simulink model "d_anderson_farmer"  (Simulink 5.1)
settings: Solver=ode45  StartTime=0.0  StopTime=10.0  RelTol=1e-3
libraries: fm_lib x1
(part 1 of 2)
settings Model: Creator=fmilano  LastModifiedBy=fmilano  ExtModeAutoUpdateStatusClock=off  SignalLoggingName=logsout  BooleanDataType=on  RTWOptions="-aEnforceIntegerDowncast=1 -aFoldNonRolledExpr=1 -aInlineInvariantSignals=0 -aInlineParameters=0 -aLocalBlockOutputs=1 -aRollThreshold=5 -aZeroInternalMemoryAtStartup=1 -aZeroExternalMemoryAtStartup=1 -aInitFltsAndDblsToZero=1 -aForceBlockIOInitOptimize=0 -aGenerateReport=0 -aGenCodeOnly=0 -aRTWVerbose=1 -aIncludeHyperlinkInReport=0 -aLaunchReport=0 -aGenerateTraceInfo=0  -aForceParamTrailComments=0 -aGenerateComments=1 -aIgnoreCustomStorageClasses=1 -aIncHierarchyInIds=0 -aMaxRTWIdLen=31 -aShowEliminatedStatements=0 -aIncDataTypeInIds=0 -aInsertBlockDesc=0 -aIgnoreTestpoints=0 -aSimulinkBlockComments=1 -aInlinedPrmAccess=\"Literals\"  -aSuppressErrorStatus=0 -aModelReferenceCompliant=1 -aParenthesesLevel=\"Nominal\" -aModelStepFunctionPrototypeControlCompliant=0 -aPortableWordSizes=0 -aParMdlRefBuildCompliant=1 -aSupportNonInlinedSFcns=1 -aSupportContinuousTime=1 -aSupportComplex=1 -aSupportNonFinite=1 -aSupportAbsoluteTime=1 -aMultiwordLength=2048 -aTargetPreCompLibLocation=\"\" -aTargetLibSuffix=\"\" -aTargetFunctionLibrary=\"ANSI_C\" -aTargetFcnLib=\"ansi_tfl_tmw.mat\" -aMultiInstanceERTCode=0 -aLogVarNameModifier=\"rt_\" -aERTFirstTimeCompliant=0 -aIsPILTarget=0 -aCombineOutputUpdateFcns=0 -aGenerateASAP2=0 -aGenerateClassInterface=0 -aGenerateTestInterfaces=0 -aGenerateSampleERTMain=0 -aGenerateFullHeader=1 -aUtilityFuncGeneration=\"Auto\" -aIncludeFileDelimiter=\"Auto\" -aIncludeMdlTerminateFcn=1 -aPurelyIntegerCode=0 -aAutosarCompliant=0 -aERTCustomFileBanners=0 -aRTWCAPIStates=0 -aRTWCAPIParams=0 -aRTWCAPISignals=0 -aMatFileLogging=1 -aCompOptLevelCompliant=0 -aCPPClassGenCompliant=0 -aExtModeIntrfLevel=\"Level1\" -aExtModeMexFile=\"ext_comm\" -aExtModeTransport=0 -aExtModeStaticAllocSize=1000000 -aExtModeTesting=0 -aExtModeStaticAlloc=0 -aExtMode=0 -aERTMultiwordLength=256 -aERTMultiwordTypeDef=\"System defined\"  -aGenerateTraceInfo=0 -aGenerateTraceInfo=0 -aGenerateTraceInfo=0 -aGenerateTraceInfo=0 -aPrefixModelToSubsysFcnNames=1"

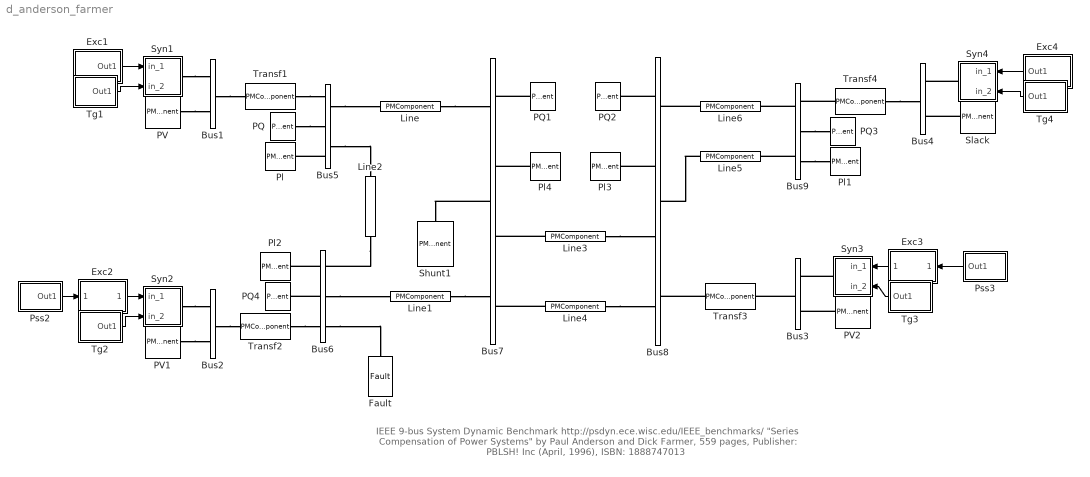
== system d_anderson_farmer ==
  note: IEEE 9-bus System Dynamic Benchmark
      |
      | http://psdyn.ece.wisc.edu/IEEE_benchmarks/
      |
      | "Series Compensation of Power Systems" by Paul Anderson and Dick Farmer,
      | 559 pages, Publisher: PBLSH! Inc (April, 1996), ISBN: 1888747013
  Bus1 : PMComponent  Tag=PSATblock  Description=Connection  PhysicalDomain=psatdomain  LeftPortType=p1  RightPortType=p1  LConnTagsString=__newl0|__newl1  RConnTagsString=__newr0  mask(Bus){in=2, out=1, p2q=20, p3_4q=[1.00   0.00], p5q=2, p6q=1}
      mask prompts: in "Number of inputs:"; out "Number of outputs:"; p2q "Voltage Rating [kV]"; p3_4q "Voltage initial guess [p.u.   rad]"; p5q "Area number"; p6q "Region number"
      mask help: Bus block
      mask init:
      | fm_inout
      settings: AttributesFormatString="|V| =  1.03   p.u.\\n<V  =  0.1540 rad"
      mask CallbackString: ||||fm_block|
      mask Display: plot([0 1 1 0 0],[0 0 1 1 0])
  Bus2 : PMComponent  Tag=PSATblock  Description=Connection  PhysicalDomain=psatdomain  LeftPortType=p1  RightPortType=p1  LConnTagsString=__newl0|__newl1  RConnTagsString=__newr0  mask(Bus){in=2, out=1, p2q=20, p3_4q=[1.00   0.00], p5q=1, p6q=1}
      mask prompts: in "Number of inputs:"; out "Number of outputs:"; p2q "Voltage Rating [kV]"; p3_4q "Voltage initial guess [p.u.   rad]"; p5q "Area number"; p6q "Region number"
      mask help: Bus block
      mask init:
      | fm_inout
      settings: AttributesFormatString="|V| =  1.05   p.u.\\n<V  =  0.1208 rad"
      mask CallbackString: ||||fm_block|
      mask Display: plot([0 1 1 0 0],[0 0 1 1 0])
  Bus3 : PMComponent  Tag=PSATblock  Description=Connection  PhysicalDomain=psatdomain  LeftPortType=p1  RightPortType=p1  LConnTagsString=__newl0  RConnTagsString=__newr0|__newr1  mask(Bus){in=1, out=2, p2q=20, p3_4q=[1.00   0.00], p5q=1, p6q=1}
      mask prompts: in "Number of inputs:"; out "Number of outputs:"; p2q "Voltage Rating [kV]"; p3_4q "Voltage initial guess [p.u.   rad]"; p5q "Area number"; p6q "Region number"
      mask help: Bus block
      mask init:
      | fm_inout
      settings: AttributesFormatString="|V| =  1.032  p.u.\\n<V  =  0.3131 rad"
      mask CallbackString: ||||fm_block|
      mask Display: plot([0 1 1 0 0],[0 0 1 1 0])
  Bus4 : PMComponent  Tag=PSATblock  Description=Connection  PhysicalDomain=psatdomain  LeftPortType=p1  RightPortType=p1  LConnTagsString=__newl0  RConnTagsString=__newr0|__newr1  mask(Bus){in=1, out=2, p2q=20, p3_4q=[1.00   0.00], p5q=3, p6q=1}
      mask prompts: in "Number of inputs:"; out "Number of outputs:"; p2q "Voltage Rating [kV]"; p3_4q "Voltage initial guess [p.u.   rad]"; p5q "Area number"; p6q "Region number"
      mask help: Bus block
      mask init:
      | fm_inout
      settings: AttributesFormatString="|V| =  1.02   p.u.\\n<V  =  0      rad"
      mask CallbackString: ||||fm_block|
      mask Display: plot([0 1 1 0 0],[0 0 1 1 0])
  Bus5 : PMComponent  Tag=PSATblock  Description=Connection  PhysicalDomain=psatdomain  LeftPortType=p1  RightPortType=p1  LConnTagsString=__newl0|__newl1|__newl2  RConnTagsString=__newr0|__newr1  mask(Bus){in=3, out=2, p2q=400, p3_4q=[1.00   0.00], p5q=2, p6q=1}
      mask prompts: in "Number of inputs:"; out "Number of outputs:"; p2q "Voltage Rating [kV]"; p3_4q "Voltage initial guess [p.u.   rad]"; p5q "Area number"; p6q "Region number"
      mask help: Bus block
      mask init:
      | fm_inout
      settings: AttributesFormatString="|V| =  1.0118 p.u.\\n<V  =  0.0752 rad"
      mask CallbackString: ||||fm_block|
      mask Display: plot([0 1 1 0 0],[0 0 1 1 0])
  Bus6 : PMComponent  Tag=PSATblock  Description=Connection  PhysicalDomain=psatdomain  LeftPortType=p1  RightPortType=p1  LConnTagsString=__newl0|__newl1|__newl2  RConnTagsString=__newr0|__newr1|__newr2  mask(Bus){in=3, out=3, p2q=400, p3_4q=[1.00   0.00], p5q=1, p6q=1}
      mask prompts: in "Number of inputs:"; out "Number of outputs:"; p2q "Voltage Rating [kV]"; p3_4q "Voltage initial guess [p.u.   rad]"; p5q "Area number"; p6q "Region number"
      mask help: Bus block
      mask init:
      | fm_inout
      settings: AttributesFormatString="|V| =  1.0397 p.u.\\n<V  =  0.0481 rad"
      mask CallbackString: ||||fm_block|
      mask Display: plot([0 1 1 0 0],[0 0 1 1 0])
  Bus7 : PMComponent  Tag=PSATblock  Description=Connection  PhysicalDomain=psatdomain  LeftPortType=p1  RightPortType=p1  LConnTagsString=__newl0|__newl1|__newl2  RConnTagsString=__newr0|__newr1|__newr2|__newr3  mask(Bus){in=3, out=4, p2q=400, p3_4q=[1.00   0.00], p5q=1, p6q=1}
      mask prompts: in "Number of inputs:"; out "Number of outputs:"; p2q "Voltage Rating [kV]"; p3_4q "Voltage initial guess [p.u.   rad]"; p5q "Area number"; p6q "Region number"
      mask help: Bus block
      mask init:
      | fm_inout
      settings: AttributesFormatString="|V| =  1.0209 p.u.\\n<V  = -0.1371 rad"
      mask CallbackString: ||||fm_block|
      mask Display: plot([0 1 1 0 0],[0 0 1 1 0])
  Bus8 : PMComponent  Tag=PSATblock  Description=Connection  PhysicalDomain=psatdomain  LeftPortType=p1  RightPortType=p1  LConnTagsString=__newl0|__newl1|__newl2|__newl3  RConnTagsString=__newr0|__newr1|__newr2  mask(Bus){in=4, out=3, p2q=400, p3_4q=[1.00   0.00], p5q=1, p6q=1}
      mask prompts: in "Number of inputs:"; out "Number of outputs:"; p2q "Voltage Rating [kV]"; p3_4q "Voltage initial guess [p.u.   rad]"; p5q "Area number"; p6q "Region number"
      mask help: Bus block
      mask init:
      | fm_inout
      settings: AttributesFormatString="|V| =  1.0247 p.u.\\n<V  =  0.2415 rad"
      mask CallbackString: ||||fm_block|
      mask Display: plot([0 1 1 0 0],[0 0 1 1 0])
  Bus9 : PMComponent  Tag=PSATblock  Description=Connection  PhysicalDomain=psatdomain  LeftPortType=p1  RightPortType=p1  LConnTagsString=__newl0|__newl1  RConnTagsString=__newr0|__newr1|__newr2  mask(Bus){in=2, out=3, p2q=400, p3_4q=[1.00   0.00], p5q=3, p6q=1}
      mask prompts: in "Number of inputs:"; out "Number of outputs:"; p2q "Voltage Rating [kV]"; p3_4q "Voltage initial guess [p.u.   rad]"; p5q "Area number"; p6q "Region number"
      mask help: Bus block
      mask init:
      | fm_inout
      settings: AttributesFormatString="|V| =  1.0005 p.u.\\n<V  = -0.0688 rad"
      mask CallbackString: ||||fm_block|
      mask Display: plot([0 1 1 0 0],[0 0 1 1 0])
  Exc1 : Subsystem  Tag=PSATblock  Description=Controls  mask(Exc){p2q=3, p3q=100, p4q=-100, p5q=100, p6q=3, p7q=1, p8q=1.00, p9q=0, p10q=0.4, p11q=0.04, p12_13q=[0.0006  0.9], in=0, p14q=on}
      mask prompts: p2q "Automatic Voltage Regulator Type"; p3q "Maximum Regulator Voltage [p.u.]"; p4q "Minimum Regulator Voltage [p.u.]"; p5q "Regulator Gain [p.u./p.u.]"; p6q "Regulator Pole T2 [s]"; p7q "Regulator Zero T1 [s]"; p8q "Second Regulator Pole T3 [s]"; p9q "Allow signal V/V0 [0 for disabling signal]"; p10q "Time Constant of the Field Circuit Td [s]"; p11q "Time Delay of the Measurement System Tr [s]"; p12_13q "Coefficient of the Ceiling Function (A B)"; in "Number of input signals"; p14q "Connected"
      mask help: This block defines an Automatic Voltage Regulator.
      mask init:
      | fm_inout
      | [x,y] = fm_draw('R');
      mask Help:
      | This block defines an Automatic Voltage Regulator.
      | There are three kind of regulators:
      | 
      | Type 1:
      | 
      |      IEEE Model 1
      | 
      | Type 2:
      | 
      |      IEEE Model 2
      | 
      | Type 3:
      | 
      |      IEEE Model 3
      mask StyleString: popup(1|2|3),edit,edit,edit,edit,edit,edit,edit,edit,edit,edit,popup(0|1|2|3),checkbox
      mask CallbackString: fm_block||||||||||||fm_block
      mask Display:
      | plot([-1.8 4.1 4.1 -1.8 -1.8],[-1.5 -1.5 1.5 1.5 -1.5])
      | color('red')
      | plot([-1.3 -0.5],[-1 1],[-0.5 0.3],[1 -1],[-0.9 -0.1],[0.0 0.0])
      | plot(2.8+1.3*x,2*y,1.5+[-1.3 -0.5],[1 -1],1.5+[-0.5 0.3],[-1 1])
  Exc2 : Subsystem  Tag=PSATblock  Description=Controls  mask(Exc){p2q=1, p3q=4, p4q=-4, p5q=200, p6q=4, p7q=1, p8q=0.006, p9q=0.06, p10q=0.0001, p11q=0.0001, p12_13q=[0.0  0.0], in=1, p14q=on}
      mask prompts: p2q "Automatic Voltage Regulator Type"; p3q "Maximum Regulator Voltage [p.u.]"; p4q "Minimum Regulator Voltage [p.u.]"; p5q "Regulator Gain m0 [p.u./p.u.]"; p6q "First Regulator Pole T1 [s]"; p7q "First Regulator Zero T2 [s]"; p8q "Second Regulator Pole T3 [s]"; p9q "Second Regulator Zero T4 [s]"; p10q "Time Constant of the Field Circuit Td [s]"; p11q "Time Delay of the Measurement System Tr [s]"; p12_13q "Coefficient of the Ceiling Function (A B)"; in "Number of input signals"; p14q "Connected"
      mask help: This block defines an Automatic Voltage Regulator.
      mask init:
      | fm_inout
      | [x,y] = fm_draw('R');
      mask Help:
      | This block defines an Automatic Voltage Regulator.
      | There are three kind of regulators:
      | 
      | Type 1:
      | 
      |      IEEE Model 1
      | 
      | Type 2:
      | 
      |      IEEE Model 2
      | 
      | Type 3:
      | 
      |      IEEE Model 3
      mask StyleString: popup(1|2|3),edit,edit,edit,edit,edit,edit,edit,edit,edit,edit,popup(0|1|2|3),checkbox
      mask CallbackString: fm_block||||||||||||fm_block
      mask Display:
      | plot([-1.8 4.1 4.1 -1.8 -1.8],[-1.5 -1.5 1.5 1.5 -1.5])
      | color('red')
      | plot([-1.3 -0.5],[-1 1],[-0.5 0.3],[1 -1],[-0.9 -0.1],[0.0 0.0])
      | plot(2.8+1.3*x,2*y,1.5+[-1.3 -0.5],[1 -1],1.5+[-0.5 0.3],[-1 1])
  Exc3 : Subsystem  Tag=PSATblock  Description=Controls  Orientation=left  mask(Exc){p2q=1, p3q=4, p4q=-4, p5q=200, p6q=4, p7q=1, p8q=0.006, p9q=0.06, p10q=0.0001, p11q=0.0001, p12_13q=[0.0  0.0], in=1, p14q=on}
      mask prompts: p2q "Automatic Voltage Regulator Type"; p3q "Maximum Regulator Voltage [p.u.]"; p4q "Minimum Regulator Voltage [p.u.]"; p5q "Regulator Gain m0 [p.u./p.u.]"; p6q "First Regulator Pole T1 [s]"; p7q "First Regulator Zero T2 [s]"; p8q "Second Regulator Pole T3 [s]"; p9q "Second Regulator Zero T4 [s]"; p10q "Time Constant of the Field Circuit Td [s]"; p11q "Time Delay of the Measurement System Tr [s]"; p12_13q "Coefficient of the Ceiling Function (A B)"; in "Number of input signals"; p14q "Connected"
      mask help: This block defines an Automatic Voltage Regulator.
      mask init:
      | fm_inout
      | [x,y] = fm_draw('R');
      mask Help:
      | This block defines an Automatic Voltage Regulator.
      | There are three kind of regulators:
      | 
      | Type 1:
      | 
      |      IEEE Model 1
      | 
      | Type 2:
      | 
      |      IEEE Model 2
      | 
      | Type 3:
      | 
      |      IEEE Model 3
      mask StyleString: popup(1|2|3),edit,edit,edit,edit,edit,edit,edit,edit,edit,edit,popup(0|1|2|3),checkbox
      mask CallbackString: fm_block||||||||||||fm_block
      mask Display:
      | plot([-1.8 4.1 4.1 -1.8 -1.8],[-1.5 -1.5 1.5 1.5 -1.5])
      | color('red')
      | plot([-1.3 -0.5],[-1 1],[-0.5 0.3],[1 -1],[-0.9 -0.1],[0.0 0.0])
      | plot(2.8+1.3*x,2*y,1.5+[-1.3 -0.5],[1 -1],1.5+[-0.5 0.3],[-1 1])
  Exc4 : Subsystem  Tag=PSATblock  Description=Controls  Orientation=left  mask(Exc){p2q=3, p3q=100, p4q=-100, p5q=100, p6q=3, p7q=1, p8q=1.00, p9q=0, p10q=0.4, p11q=0.04, p12_13q=[0.0006  0.9], in=0, p14q=on}
      mask prompts: p2q "Automatic Voltage Regulator Type"; p3q "Maximum Regulator Voltage [p.u.]"; p4q "Minimum Regulator Voltage [p.u.]"; p5q "Regulator Gain [p.u./p.u.]"; p6q "Regulator Pole T2 [s]"; p7q "Regulator Zero T1 [s]"; p8q "Second Regulator Pole T3 [s]"; p9q "Allow signal V/V0 [0 for disabling signal]"; p10q "Time Constant of the Field Circuit Td [s]"; p11q "Time Delay of the Measurement System Tr [s]"; p12_13q "Coefficient of the Ceiling Function (A B)"; in "Number of input signals"; p14q "Connected"
      mask help: This block defines an Automatic Voltage Regulator.
      mask init:
      | fm_inout
      | [x,y] = fm_draw('R');
      mask Help:
      | This block defines an Automatic Voltage Regulator.
      | There are three kind of regulators:
      | 
      | Type 1:
      | 
      |      IEEE Model 1
      | 
      | Type 2:
      | 
      |      IEEE Model 2
      | 
      | Type 3:
      | 
      |      IEEE Model 3
      mask StyleString: popup(1|2|3),edit,edit,edit,edit,edit,edit,edit,edit,edit,edit,popup(0|1|2|3),checkbox
      mask CallbackString: fm_block||||||||||||fm_block
      mask Display:
      | plot([-1.8 4.1 4.1 -1.8 -1.8],[-1.5 -1.5 1.5 1.5 -1.5])
      | color('red')
      | plot([-1.3 -0.5],[-1 1],[-0.5 0.3],[1 -1],[-0.9 -0.1],[0.0 0.0])
      | plot(2.8+1.3*x,2*y,1.5+[-1.3 -0.5],[1 -1],1.5+[-0.5 0.3],[-1 1])
  Fault : fm_lib/Faults &  Breakers/Fault  Tag=PSATblock  Description=Faults & Breakers  Orientation=down  PhysicalDomain=psatdomain  SubClassName=unknown  LeftPortType=p1  RightPortType=p1  LConnTagsString=__newl0  p2_3_4q="[100  400  60]"  p5q=0.00  p6q=4/60  p7q=0  p8q=1e-6
  Line : PMComponent  Tag=PSATblock  Description=Power Flow  PhysicalDomain=psatdomain  LeftPortType=p1  RightPortType=p1  LConnTagsString=__newl0  RConnTagsString=__newr0  mask(Line){p3_4_5q=[100  400  60], p6q=0, p8q=0.003618, p9q=0.024241, p10q=1.767004, p13_14_15q=[0.0  0.0  0.0], p16q=on}
      mask prompts: p3_4_5q "Power, Voltage and Frequency Ratings [MVA, kV, Hz]"; p6q "Length of line [km] (0 for p.u. parameters)"; p8q "Resistance [p.u. (Ohms/km)]"; p9q "Reactance [p.u. (H/km)]"; p10q "Susceptance [p.u. (F/km)]"; p13_14_15q "Imax, Pmax and Smax [p.u., p.u., p.u.]"; p16q "Connected"
      mask help: This block defines a pi model for a tree phase line.
      mask init:
      | [xp,yp] = fm_draw('pi');
      mask CallbackString: ||||||fm_block
      mask Display:
      | plot([-1  1  1 -1 -1],[-0.2 -0.2 0.2 0.2 -0.2])
      | color('blue')
      | plot(0.35*xp,0.2*yp)
  Line1 : PMComponent  Tag=PSATblock  Description=Power Flow  PhysicalDomain=psatdomain  LeftPortType=p1  RightPortType=p1  LConnTagsString=__newl0  RConnTagsString=__newr0  mask(Line){p3_4_5q=[100  400  60], p6q=0, p8q=0.003618, p9q=0.024241, p10q=1.767004, p13_14_15q=[0.0  0.0  0.0], p16q=on}
      mask prompts: p3_4_5q "Power, Voltage and Frequency Ratings [MVA, kV, Hz]"; p6q "Length of line [km] (0 for p.u. parameters)"; p8q "Resistance [p.u. (Ohms/km)]"; p9q "Reactance [p.u. (H/km)]"; p10q "Susceptance [p.u. (F/km)]"; p13_14_15q "Imax, Pmax and Smax [p.u., p.u., p.u.]"; p16q "Connected"
      mask help: This block defines a pi model for a tree phase line.
      mask init:
      | [xp,yp] = fm_draw('pi');
      mask CallbackString: ||||||fm_block
      mask Display:
      | plot([-1  1  1 -1 -1],[-0.2 -0.2 0.2 0.2 -0.2])
      | color('blue')
      | plot(0.35*xp,0.2*yp)
  Line2 : PMComponent  Tag=PSATblock  Description=Power Flow  Orientation=down  PhysicalDomain=psatdomain  LeftPortType=p1  RightPortType=p1  LConnTagsString=__newl0  RConnTagsString=__newr0  mask(Line){p3_4_5q=[100  400  60], p6q=0, p8q=0.003226, p9q=0.020851, p10q=1.449019, p13_14_15q=[0.0  0.0  0.0], p16q=on}
      mask prompts: p3_4_5q "Power, Voltage and Frequency Ratings [MVA, kV, Hz]"; p6q "Length of line [km] (0 for p.u. parameters)"; p8q "Resistance [p.u. (Ohms/km)]"; p9q "Reactance [p.u. (H/km)]"; p10q "Susceptance [p.u. (F/km)]"; p13_14_15q "Imax, Pmax and Smax [p.u., p.u., p.u.]"; p16q "Connected"
      mask help: This block defines a pi model for a tree phase line.
      mask init:
      | [xp,yp] = fm_draw('pi');
      mask CallbackString: ||||||fm_block
      mask Display:
      | plot([-1  1  1 -1 -1],[-0.2 -0.2 0.2 0.2 -0.2])
      | color('blue')
      | plot(0.35*xp,0.2*yp)
  Line3 : PMComponent  Tag=PSATblock  Description=Power Flow  PhysicalDomain=psatdomain  LeftPortType=p1  RightPortType=p1  LConnTagsString=__newl0  RConnTagsString=__newr0  mask(Line){p3_4_5q=[100  400  60], p6q=0, p8q=0.003226, p9q=0.069502, p10q=1.449019, p13_14_15q=[0.0  0.0  0.0], p16q=on}
      mask prompts: p3_4_5q "Power, Voltage and Frequency Ratings [MVA, kV, Hz]"; p6q "Length of line [km] (0 for p.u. parameters)"; p8q "Resistance [p.u. (Ohms/km)]"; p9q "Reactance [p.u. (H/km)]"; p10q "Susceptance [p.u. (F/km)]"; p13_14_15q "Imax, Pmax and Smax [p.u., p.u., p.u.]"; p16q "Connected"
      mask help: This block defines a pi model for a tree phase line.
      mask init:
      | [xp,yp] = fm_draw('pi');
      mask CallbackString: ||||||fm_block
      mask Display:
      | plot([-1  1  1 -1 -1],[-0.2 -0.2 0.2 0.2 -0.2])
      | color('blue')
      | plot(0.35*xp,0.2*yp)
  Line4 : PMComponent  Tag=PSATblock  Description=Power Flow  PhysicalDomain=psatdomain  LeftPortType=p1  RightPortType=p1  LConnTagsString=__newl0  RConnTagsString=__newr0  mask(Line){p3_4_5q=[100  400  60], p6q=0, p8q=0.003226, p9q=0.069502, p10q=1.449019, p13_14_15q=[0.0  0.0  0.0], p16q=on}
      mask prompts: p3_4_5q "Power, Voltage and Frequency Ratings [MVA, kV, Hz]"; p6q "Length of line [km] (0 for p.u. parameters)"; p8q "Resistance [p.u. (Ohms/km)]"; p9q "Reactance [p.u. (H/km)]"; p10q "Susceptance [p.u. (F/km)]"; p13_14_15q "Imax, Pmax and Smax [p.u., p.u., p.u.]"; p16q "Connected"
      mask help: This block defines a pi model for a tree phase line.
      mask init:
      | [xp,yp] = fm_draw('pi');
      mask CallbackString: ||||||fm_block
      mask Display:
      | plot([-1  1  1 -1 -1],[-0.2 -0.2 0.2 0.2 -0.2])
      | color('blue')
      | plot(0.35*xp,0.2*yp)
  Line5 : PMComponent  Tag=PSATblock  Description=Power Flow  PhysicalDomain=psatdomain  LeftPortType=p1  RightPortType=p1  LConnTagsString=__newl0  RConnTagsString=__newr0  mask(Line){p3_4_5q=[100  400  60], p6q=0, p8q=0.003226, p9q=0.069502, p10q=1.449019, p13_14_15q=[0.0  0.0  0.0], p16q=on}
      mask prompts: p3_4_5q "Power, Voltage and Frequency Ratings [MVA, kV, Hz]"; p6q "Length of line [km] (0 for p.u. parameters)"; p8q "Resistance [p.u. (Ohms/km)]"; p9q "Reactance [p.u. (H/km)]"; p10q "Susceptance [p.u. (F/km)]"; p13_14_15q "Imax, Pmax and Smax [p.u., p.u., p.u.]"; p16q "Connected"
      mask help: This block defines a pi model for a tree phase line.
      mask init:
      | [xp,yp] = fm_draw('pi');
      mask CallbackString: ||||||fm_block
      mask Display:
      | plot([-1  1  1 -1 -1],[-0.2 -0.2 0.2 0.2 -0.2])
      | color('blue')
      | plot(0.35*xp,0.2*yp)
  Line6 : PMComponent  Tag=PSATblock  Description=Power Flow  PhysicalDomain=psatdomain  LeftPortType=p1  RightPortType=p1  LConnTagsString=__newl0  RConnTagsString=__newr0  mask(Line){p3_4_5q=[100  400  60], p6q=0, p8q=0.003226, p9q=0.069502, p10q=1.449019, p13_14_15q=[0.0  0.0  0.0], p16q=on}
      mask prompts: p3_4_5q "Power, Voltage and Frequency Ratings [MVA, kV, Hz]"; p6q "Length of line [km] (0 for p.u. parameters)"; p8q "Resistance [p.u. (Ohms/km)]"; p9q "Reactance [p.u. (H/km)]"; p10q "Susceptance [p.u. (F/km)]"; p13_14_15q "Imax, Pmax and Smax [p.u., p.u., p.u.]"; p16q "Connected"
      mask help: This block defines a pi model for a tree phase line.
      mask init:
      | [xp,yp] = fm_draw('pi');
      mask CallbackString: ||||||fm_block
      mask Display:
      | plot([-1  1  1 -1 -1],[-0.2 -0.2 0.2 0.2 -0.2])
      | color('blue')
      | plot(0.35*xp,0.2*yp)
  PQ : PMComponent  Tag=PSATblock  Description=Power Flow  Orientation=left  PhysicalDomain=psatdomain  LeftPortType=p1  RightPortType=p1  LConnTagsString=__newl0  mask(PQ){p2_3q=[100  400], p4_5q=[400  80], p6_7q=[1.2  0.8], p8q=on, p9q=on}
      mask prompts: p2_3q "Power and Voltage Ratings [MVA, kV]"; p4_5q "Active and Reactive Powers [p.u.  p.u.]"; p6_7q "Maximum and Minimum Allowable Voltage [p.u.   p.u.]"; p8q "Allow conversion to impendance for min or max voltage"; p9q "Connected"
      mask help:
      | This block defines a constant power load:
      |
      | P = Pcost.
      | Q = Qcost.
      mask CallbackString: |||fm_block|fm_block
      mask Display: plot([1 -0.5 -0.5 1],[0 0.866 -0.866 0])
  PQ1 : PMComponent  Tag=PSATblock  Description=Power Flow  PhysicalDomain=psatdomain  LeftPortType=p1  RightPortType=p1  LConnTagsString=__newl0  mask(PQ){p2_3q=[100  400], p4_5q=[27.5  5.50], p6_7q=[1.2  0.8], p8q=on, p9q=on}
      mask prompts: p2_3q "Power and Voltage Ratings [MVA, kV]"; p4_5q "Active and Reactive Powers [p.u.  p.u.]"; p6_7q "Maximum and Minimum Allowable Voltage [p.u.   p.u.]"; p8q "Allow conversion to impendance for min or max voltage"; p9q "Connected"
      mask help:
      | This block defines a constant power load:
      |
      | P = Pcost.
      | Q = Qcost.
      mask CallbackString: |||fm_block|fm_block
      mask Display: plot([1 -0.5 -0.5 1],[0 0.866 -0.866 0])
  PQ2 : PMComponent  Tag=PSATblock  Description=Power Flow  Orientation=left  PhysicalDomain=psatdomain  LeftPortType=p1  RightPortType=p1  LConnTagsString=__newl0  mask(PQ){p2_3q=[100  400], p4_5q=[17.5  2], p6_7q=[1.2  0.8], p8q=on, p9q=on}
      mask prompts: p2_3q "Power and Voltage Ratings [MVA, kV]"; p4_5q "Active and Reactive Powers [p.u.  p.u.]"; p6_7q "Maximum and Minimum Allowable Voltage [p.u.   p.u.]"; p8q "Allow conversion to impendance for min or max voltage"; p9q "Connected"
      mask help:
      | This block defines a constant power load:
      |
      | P = Pcost.
      | Q = Qcost.
      mask CallbackString: |||fm_block|fm_block
      mask Display: plot([1 -0.5 -0.5 1],[0 0.866 -0.866 0])
  PQ3 : PMComponent  Tag=PSATblock  Description=Power Flow  PhysicalDomain=psatdomain  LeftPortType=p1  RightPortType=p1  LConnTagsString=__newl0  mask(PQ){p2_3q=[100  400], p4_5q=[500  120], p6_7q=[1.2  0.8], p8q=on, p9q=on}
      mask prompts: p2_3q "Power and Voltage Ratings [MVA, kV]"; p4_5q "Active and Reactive Powers [p.u.  p.u.]"; p6_7q "Maximum and Minimum Allowable Voltage [p.u.   p.u.]"; p8q "Allow conversion to impendance for min or max voltage"; p9q "Connected"
      mask help:
      | This block defines a constant power load:
      |
      | P = Pcost.
      | Q = Qcost.
      mask CallbackString: |||fm_block|fm_block
      mask Display: plot([1 -0.5 -0.5 1],[0 0.866 -0.866 0])
  PQ4 : PMComponent  Tag=PSATblock  Description=Power Flow  Orientation=left  PhysicalDomain=psatdomain  LeftPortType=p1  RightPortType=p1  LConnTagsString=__newl0  mask(PQ){p2_3q=[100  400], p4_5q=[5  1], p6_7q=[1.2  0.8], p8q=on, p9q=on}
      mask prompts: p2_3q "Power and Voltage Ratings [MVA, kV]"; p4_5q "Active and Reactive Powers [p.u.  p.u.]"; p6_7q "Maximum and Minimum Allowable Voltage [p.u.   p.u.]"; p8q "Allow conversion to impendance for min or max voltage"; p9q "Connected"
      mask help:
      | This block defines a constant power load:
      |
      | P = Pcost.
      | Q = Qcost.
      mask CallbackString: |||fm_block|fm_block
      mask Display: plot([1 -0.5 -0.5 1],[0 0.866 -0.866 0])
  PV : PMComponent  Tag=PSATblock  Description=Power Flow  PhysicalDomain=psatdomain  LeftPortType=p1  RightPortType=p1  RConnTagsString=__newr0  mask(PV){p2_3q=[100  20], p4q=410, p5q=1.03, p6_7q=[0.8  -0.2], p8_9q=[1.1  0.9], p10q=1, p11q=on}
      mask prompts: p2_3q "Power and Voltage Ratings [MVA, kV]"; p4q "Active Power [p.u.]"; p5q "Voltage Magnitude [p.u.]"; p6_7q "Qmax and Qmin [p.u.  p.u.]"; p8_9q "Vmax and Vmin [p.u.  p.u.]"; p10q "Loss Participation Factor"; p11q "Connected"
      mask help:
      | This block defines a PV bus for load flow studies:
      |
      | P = Pcost.
      | V = Vdes.
      mask init:
      | [x,y] = fm_draw('circle');
      | [xp,yp] = fm_draw('P');
      mask CallbackString: ||||||fm_block
      mask Display:
      | plot(x,y)
      | color('blue')
      | plot(0.3*xp-0.35,0.6*yp,[0.1 0.3 0.5],[0.3 -0.3 0.3])
  PV1 : PMComponent  Tag=PSATblock  Description=Power Flow  PhysicalDomain=psatdomain  LeftPortType=p1  RightPortType=p1  RConnTagsString=__newr0  mask(PV){p2_3q=[100  20], p4q=12, p5q=1.05, p6_7q=[0.8  -0.2], p8_9q=[1.1  0.9], p10q=1, p11q=on}
      mask prompts: p2_3q "Power and Voltage Ratings [MVA, kV]"; p4q "Active Power [p.u.]"; p5q "Voltage Magnitude [p.u.]"; p6_7q "Qmax and Qmin [p.u.  p.u.]"; p8_9q "Vmax and Vmin [p.u.  p.u.]"; p10q "Loss Participation Factor"; p11q "Connected"
      mask help:
      | This block defines a PV bus for load flow studies:
      |
      | P = Pcost.
      | V = Vdes.
      mask init:
      | [x,y] = fm_draw('circle');
      | [xp,yp] = fm_draw('P');
      mask CallbackString: ||||||fm_block
      mask Display:
      | plot(x,y)
      | color('blue')
      | plot(0.3*xp-0.35,0.6*yp,[0.1 0.3 0.5],[0.3 -0.3 0.3])
  PV2 : PMComponent  Tag=PSATblock  Description=Power Flow  Orientation=left  PhysicalDomain=psatdomain  LeftPortType=p1  RightPortType=p1  RConnTagsString=__newr0  mask(PV){p2_3q=[100  20], p4q=37.801, p5q=1.032, p6_7q=[0.8  -0.2], p8_9q=[1.1  0.9], p10q=1, p11q=on}
      mask prompts: p2_3q "Power and Voltage Ratings [MVA, kV]"; p4q "Active Power [p.u.]"; p5q "Voltage Magnitude [p.u.]"; p6_7q "Qmax and Qmin [p.u.  p.u.]"; p8_9q "Vmax and Vmin [p.u.  p.u.]"; p10q "Loss Participation Factor"; p11q "Connected"
      mask help:
      | This block defines a PV bus for load flow studies:
      |
      | P = Pcost.
      | V = Vdes.
      mask init:
      | [x,y] = fm_draw('circle');
      | [xp,yp] = fm_draw('P');
      mask CallbackString: ||||||fm_block
      mask Display:
      | plot(x,y)
      | color('blue')
      | plot(0.3*xp-0.35,0.6*yp,[0.1 0.3 0.5],[0.3 -0.3 0.3])
  Pl : PMComponent  Tag=PSATblock  Description=Loads  Orientation=left  PhysicalDomain=psatdomain  LeftPortType=p1  RightPortType=p1  LConnTagsString=__newl0  mask(Pl){p2_3_4q=[100 400 60], p5_6_7q=[0 0 100], p8_9_10q=[0 0 100], p11q=on, p12q=on}
      mask prompts: p2_3_4q "Power, voltage and frequency ratings [MVA, kV, Hz]"; p5_6_7q "Percentage of resistance, active current and active power [%, %, %]"; p8_9_10q "Percentage of reactance, reactive current and reactive power [%, %, %]"; p11q "Initialize after power flow"; p12q "Connected"
      mask help: This block defines a ZIP load.
      mask CallbackString: |||fm_block|fm_block
      mask Display:
      | plot([-1 -1 1 1 -1],[-1 1 1 -1 -1])
      | color('blue')
      | plot([0 0],[-0.3 0.3],[-0.3 -0.7 -0.3 -0.7],[-0.3 -0.3 0.3 0.3])
      | plot([0.3 0.3 0.6 0.7 0.7 0.6 0.3],[-0.3 0.3 0.3 0.2 0.1 0 0])
  Pl1 : PMComponent  Tag=PSATblock  Description=Loads  PhysicalDomain=psatdomain  LeftPortType=p1  RightPortType=p1  LConnTagsString=__newl0  mask(Pl){p2_3_4q=[100 400 60], p5_6_7q=[0 0 100], p8_9_10q=[0 0 100], p11q=on, p12q=on}
      mask prompts: p2_3_4q "Power, voltage and frequency ratings [MVA, kV, Hz]"; p5_6_7q "Percentage of resistance, active current and active power [%, %, %]"; p8_9_10q "Percentage of reactance, reactive current and reactive power [%, %, %]"; p11q "Initialize after power flow"; p12q "Connected"
      mask help: This block defines a ZIP load.
      mask CallbackString: |||fm_block|fm_block
      mask Display:
      | plot([-1 -1 1 1 -1],[-1 1 1 -1 -1])
      | color('blue')
      | plot([0 0],[-0.3 0.3],[-0.3 -0.7 -0.3 -0.7],[-0.3 -0.3 0.3 0.3])
      | plot([0.3 0.3 0.6 0.7 0.7 0.6 0.3],[-0.3 0.3 0.3 0.2 0.1 0 0])
  Pl2 : PMComponent  Tag=PSATblock  Description=Loads  Orientation=left  PhysicalDomain=psatdomain  LeftPortType=p1  RightPortType=p1  LConnTagsString=__newl0  mask(Pl){p2_3_4q=[100 400 60], p5_6_7q=[0 100 0], p8_9_10q=[0 100 0], p11q=on, p12q=on}
      mask prompts: p2_3_4q "Power, voltage and frequency ratings [MVA, kV, Hz]"; p5_6_7q "Percentage of resistance, active current and active power [%, %, %]"; p8_9_10q "Percentage of reactance, reactive current and reactive power [%, %, %]"; p11q "Initialize after power flow"; p12q "Connected"
      mask help: This block defines a ZIP load.
      mask CallbackString: |||fm_block|fm_block
      mask Display:
      | plot([-1 -1 1 1 -1],[-1 1 1 -1 -1])
      | color('blue')
      | plot([0 0],[-0.3 0.3],[-0.3 -0.7 -0.3 -0.7],[-0.3 -0.3 0.3 0.3])
      | plot([0.3 0.3 0.6 0.7 0.7 0.6 0.3],[-0.3 0.3 0.3 0.2 0.1 0 0])
  Pl3 : PMComponent  Tag=PSATblock  Description=Loads  Orientation=left  PhysicalDomain=psatdomain  LeftPortType=p1  RightPortType=p1  LConnTagsString=__newl0  mask(Pl){p2_3_4q=[100 400 60], p5_6_7q=[0 100 0], p8_9_10q=[0 100 0], p11q=on, p12q=on}
      mask prompts: p2_3_4q "Power, voltage and frequency ratings [MVA, kV, Hz]"; p5_6_7q "Percentage of resistance, active current and active power [%, %, %]"; p8_9_10q "Percentage of reactance, reactive current and reactive power [%, %, %]"; p11q "Initialize after power flow"; p12q "Connected"
      mask help: This block defines a ZIP load.
      mask CallbackString: |||fm_block|fm_block
      mask Display:
      | plot([-1 -1 1 1 -1],[-1 1 1 -1 -1])
      | color('blue')
      | plot([0 0],[-0.3 0.3],[-0.3 -0.7 -0.3 -0.7],[-0.3 -0.3 0.3 0.3])
      | plot([0.3 0.3 0.6 0.7 0.7 0.6 0.3],[-0.3 0.3 0.3 0.2 0.1 0 0])
  Pl4 : PMComponent  Tag=PSATblock  Description=Loads  PhysicalDomain=psatdomain  LeftPortType=p1  RightPortType=p1  LConnTagsString=__newl0  mask(Pl){p2_3_4q=[100 400 60], p5_6_7q=[0 100 0], p8_9_10q=[0 100 0], p11q=on, p12q=on}
      mask prompts: p2_3_4q "Power, voltage and frequency ratings [MVA, kV, Hz]"; p5_6_7q "Percentage of resistance, active current and active power [%, %, %]"; p8_9_10q "Percentage of reactance, reactive current and reactive power [%, %, %]"; p11q "Initialize after power flow"; p12q "Connected"
      mask help: This block defines a ZIP load.
      mask CallbackString: |||fm_block|fm_block
      mask Display:
      | plot([-1 -1 1 1 -1],[-1 1 1 -1 -1])
      | color('blue')
      | plot([0 0],[-0.3 0.3],[-0.3 -0.7 -0.3 -0.7],[-0.3 -0.3 0.3 0.3])
      | plot([0.3 0.3 0.6 0.7 0.7 0.6 0.3],[-0.3 0.3 0.3 0.2 0.1 0 0])
  Pss2 : Subsystem  Tag=PSATblock  Description=Controls  mask(Pss){p2q=2, p3q=omega, p4_5q=[0.1 -0.1], p6_7q=[15  10], p14_15q=20  5, p8_9_10_11q=[0.1 0.01 0.12 0.01], p12_13q=[25 0.5], p16_17_18_19q=[0.045  0.045  0.045  -0.045], p20_21q=[1.000  0.95], p22q=off, p23q=on}
      mask prompts: p2q "PSS model"; p3q "Input Signal"; p4_5q "Max and Min Stabilizer Output [p.u.]"; p6_7q "Gain Kw and time constant Tw  [p.u./p.u., s]"; p14_15q "Electrical power gain Kp and voltage gain Kv [p.u./p.u., p.u./p.u.]"; p8_9_10_11q "Lead-Lag time constants T1, T2, T3, T4 [s, s, s, s]"; p12_13q "Gain Ka and time constant Ta [p.u./p.u., s]"; p16_17_18_19q "Additional signal limits Va_max, Va_thr, V3_max and V3_min [p.u., p.u., p.u., p.u.]"; p20_21q "Threshold limits E_thr and w_thr [p.u., p.u.]"; p22q "Allow switch S2"; p23q "Connected"
      mask help: This block defines a Power System Stabilizer.
      mask init:
      | [xs,ys] = fm_draw('S');
      | [xp,yp] = fm_draw('P');
      mask StyleString: popup(1|2|3|4|5),popup(omega|power|voltage),edit,edit,edit,edit,edit,edit,edit,checkbox,checkbox
      mask CallbackString: fm_block||||||||||fm_block
      mask Display:
      | plot([-1.8 4.1 4.1 -1.8 -1.8],[-1.5 -1.5 1.5 1.5 -1.5])
      | color('red')
      | plot(1.5*xp-0.7,2*yp,1.2+1.5*xs,2*ys,2.8+1.5*xs,2*ys)
  Pss3 : Subsystem  Tag=PSATblock  Description=Controls  Orientation=left  mask(Pss){p2q=2, p3q=omega, p4_5q=[0.1 -0.1], p6_7q=[20  10], p14_15q=20  5, p8_9_10_11q=[0.1 0.01 0.12 0.01], p12_13q=[25 0.5], p16_17_18_19q=[0.045  0.045  0.045  -0.045], p20_21q=[1.000  0.95], p22q=off, p23q=on}
      mask prompts: p2q "PSS model"; p3q "Input Signal"; p4_5q "Max and Min Stabilizer Output [p.u.]"; p6_7q "Gain Kw and time constant Tw  [p.u./p.u., s]"; p14_15q "Electrical power gain Kp and voltage gain Kv [p.u./p.u., p.u./p.u.]"; p8_9_10_11q "Lead-Lag time constants T1, T2, T3, T4 [s, s, s, s]"; p12_13q "Gain Ka and time constant Ta [p.u./p.u., s]"; p16_17_18_19q "Additional signal limits Va_max, Va_thr, V3_max and V3_min [p.u., p.u., p.u., p.u.]"; p20_21q "Threshold limits E_thr and w_thr [p.u., p.u.]"; p22q "Allow switch S2"; p23q "Connected"
      mask help: This block defines a Power System Stabilizer.
      mask init:
      | [xs,ys] = fm_draw('S');
      | [xp,yp] = fm_draw('P');
      mask StyleString: popup(1|2|3|4|5),popup(omega|power|voltage),edit,edit,edit,edit,edit,edit,edit,checkbox,checkbox
      mask CallbackString: fm_block||||||||||fm_block
      mask Display:
      | plot([-1.8 4.1 4.1 -1.8 -1.8],[-1.5 -1.5 1.5 1.5 -1.5])
      | color('red')
      | plot(1.5*xp-0.7,2*yp,1.2+1.5*xs,2*ys,2.8+1.5*xs,2*ys)
  Shunt1 : PMComponent  Tag=PSATblock  Description=Power Flow  Orientation=down  PhysicalDomain=psatdomain  LeftPortType=p1  RightPortType=p1  LConnTagsString=__newl0  mask(Shunt){p2_3_4q=[100  400  60], p6q=1/0.123457, p7q=on}
      mask prompts: p2_3_4q "Power, Voltage and Frequency Ratings [MVA, kV, Hz]"; p6q "Susceptance B [p.u.]"; p7q "Connected"
      mask help:
      | This block defines a static condenser:
      |
      | Q = B * V^2
      |
      | (Negative values of B define an inductive load).
      mask init:
      | fm_block
      mask CallbackString: ||fm_block
      mask Display: plot(-[0 60 60 55 53 55 60 60 55 53]/150,[0 0 8 16 25 16 8 -8 -16 -25]/50,-[80 80 80 150]/150,[25 -25 0 0]/50,[0 0],[-0.4 0.4],[0.075 0.075],[-0.25 0.25],[0.15 0.15],[-0.1 0.1])
  Slack : PMComponent  Tag=PSATblock  Description=Power Flow  Orientation=left  PhysicalDomain=psatdomain  LeftPortType=p1  RightPortType=p1  RConnTagsString=__newr0  mask(SW){p2_3q=[100  20], p4q=1.02, p5q=0.00, p6_7q=[1.5  -1.5], p8_9q=[1.1  0.9], p10q=0.80, p11q=1, p12q=on, p13q=on}
      mask prompts: p2_3q "Power and Voltage Ratings [MVA, kV]"; p4q "Voltage Magnitude [p.u.]"; p5q "Reference Phase Angle [rad]"; p6_7q "Qmax and Qmin [p.u.  p.u.]"; p8_9q "Vmax and Vmin  [p.u.  p.u.]"; p10q "Active Power Guess [p.u.]"; p11q "Loss Participation Factor"; p12q "Reference bus"; p13q "Connected"
      mask help:
      | This block defines a V-theta bus:
      |
      | V = V_des
      | theta = theta_des
      mask init:
      | [x,y] = fm_draw('circle');
      | [xt,yt] = fm_draw('theta');
      mask CallbackString: |||||||fm_block|fm_block
      mask Display: plot([0 1 1 0 0],[0 0 1 1 0]), color('blue'), plot([0 1],[0 1],[0 1],[1 0],[0.5 1 0.5 0 0.5],[0 0.5 1 0.5 0])
  Syn1 : Subsystem  Tag=PSATblock  Description=Machines  mask(Syn){p2_3_4q=[60000  20   60], p5q=2, p7_6q=[0.0046  0*0.155], p8_9_10q=[2.11  0.28  0.215], p11_12q=[4.2  0.032], p13_14_15q=[2.02  0.49  0.215], p16_17q=[0.565  0.062], p18_19q=[2*2.318  2.00], p20_21q=[0.00  0.00], p22_23q=[1.00  1.00], p24q=0.00, p25_26q=[0 0], in=2, p27q=1, p28q=on}
      mask prompts: p2_3_4q "Power, voltage and frequency ratings [MVA, kV, Hz]"; p5q "Machine Dynamic Order"; p7_6q "resistance ra and leakage reactance xl [p.u. p.u.]"; p8_9_10q "d-axis reactances Xd, X'd X"d [p.u.,p.u.,p.u.]"; p11_12q "d-axis open circuit time constants T'd0 and T"d0 [s, s]"; p13_14_15q "q-axis reactances Xq, X'q, X"q [p.u.  p.u.  p.u.]"; p16_17q "q-axis open circuit time constants T'q0 and T"q0 [s s]"; p18_19q "Inertia (M = 2H) and Damping [s, p.u.]"; p20_21q "Speed and active power additional signals Kw and Kp [p.u., p.u.]"; p22_23q "Percentage of active and reactive powers at bus [p.u. p.u.]"; p24q "d-axis additional circuit leakage time constant Taa [s]"; p25_26q "Saturation coefficients S(1.0) and S(1.2)"; in "Number of input signals"; p27q "COI number"; p28q "Connected"
      mask help: This block defines a fourth order synchronous machine.
      mask init:
      | fm_inout
      | [x,y] = fm_draw('circle');
      | [xg,yg] = fm_draw('G');
      | [xs,ys] = fm_draw('sinus');
      mask StyleString: edit,popup(8|6|5.3|5.2|5.1|4|3|2),edit,edit,edit,edit,edit,edit,edit,edit,edit,edit,popup(0|1|2),edit,checkbox
      mask CallbackString: |fm_block|||||||||||||fm_block
      mask Display:
      | plot(x+1.4,y,0.12*xs+1,0.15*ys-0.6)
      | color('blue')
      | plot(1.4+0.45*xg,0.3+0.45*yg)
  Syn2 : Subsystem  Tag=PSATblock  Description=Machines  mask(Syn){p2_3_4q=[1300  20   60], p5q=6, p7_6q=[0.0019  0*0.246], p8_9_10q=[2.183  0.413  0.339], p11_12q=[5.690  0.041], p13_14_15q=[2.157  1.285  0.332], p16_17q=[1.5  0.144], p18_19q=[2*2.642  2.00], p20_21q=[0.00  0.00], p22_23q=[1.00  1.00], p24q=0.00, p25_26q=[0 0], in=2, p27q=1, p28q=on}
      mask prompts: p2_3_4q "Power, voltage and frequency ratings [MVA, kV, Hz]"; p5q "Machine Dynamic Order"; p7_6q "resistance ra and leakage reactance xl [p.u. p.u.]"; p8_9_10q "d-axis reactances Xd, X'd X"d [p.u.,p.u.,p.u.]"; p11_12q "d-axis open circuit time constants T'd0 and T"d0 [s, s]"; p13_14_15q "q-axis reactances Xq, X'q, X"q [p.u.  p.u.  p.u.]"; p16_17q "q-axis open circuit time constants T'q0 and T"q0 [s s]"; p18_19q "Inertia (M = 2H) and Damping [s, p.u.]"; p20_21q "Speed and active power additional signals Kw and Kp [p.u., p.u.]"; p22_23q "Percentage of active and reactive powers at bus [p.u. p.u.]"; p24q "d-axis additional circuit leakage time constant Taa [s]"; p25_26q "Saturation coefficients S(1.0) and S(1.2)"; in "Number of input signals"; p27q "COI number"; p28q "Connected"
      mask help: This block defines a fourth order synchronous machine.
      mask init:
      | fm_inout
      | [x,y] = fm_draw('circle');
      | [xg,yg] = fm_draw('G');
      | [xs,ys] = fm_draw('sinus');
      mask StyleString: edit,popup(8|6|5.3|5.2|5.1|4|3|2),edit,edit,edit,edit,edit,edit,edit,edit,edit,edit,popup(0|1|2),edit,checkbox
      mask CallbackString: |fm_block|||||||||||||fm_block
      mask Display:
      | plot(x+1.4,y,0.12*xs+1,0.15*ys-0.6)
      | color('blue')
      | plot(1.4+0.45*xg,0.3+0.45*yg)
  Syn3 : Subsystem  Tag=PSATblock  Description=Machines  Orientation=left  mask(Syn){p2_3_4q=[4400  20   60], p5q=6, p7_6q=[0.0031  0*0.11], p8_9_10q=[1.70  0.245  0.185], p11_12q=[5.9  0.033], p13_14_15q=[1.64  0.38  0.185], p16_17q=[0.54  0.076], p18_19q=[2*3.96  2.00], p20_21q=[0.00  0.00], p22_23q=[1.00  1.00], p24q=0.0, p25_26q=[0 0], in=2, p27q=1, p28q=on}
      mask prompts: p2_3_4q "Power, voltage and frequency ratings [MVA, kV, Hz]"; p5q "Machine Dynamic Order"; p7_6q "resistance ra and leakage reactance xl [p.u. p.u.]"; p8_9_10q "d-axis reactances Xd, X'd X"d [p.u.,p.u.,p.u.]"; p11_12q "d-axis open circuit time constants T'd0 and T"d0 [s, s]"; p13_14_15q "q-axis reactances Xq, X'q, X"q [p.u.  p.u.  p.u.]"; p16_17q "q-axis open circuit time constants T'q0 and T"q0 [s s]"; p18_19q "Inertia (M = 2H) and Damping [s, p.u.]"; p20_21q "Speed and active power additional signals Kw and Kp [p.u., p.u.]"; p22_23q "Percentage of active and reactive powers at bus [p.u. p.u.]"; p24q "d-axis additional circuit leakage time constant Taa [s]"; p25_26q "Saturation coefficients S(1.0) and S(1.2)"; in "Number of input signals"; p27q "COI number"; p28q "Connected"
      mask help: This block defines a fourth order synchronous machine.
      mask init:
      | fm_inout
      | [x,y] = fm_draw('circle');
      | [xg,yg] = fm_draw('G');
      | [xs,ys] = fm_draw('sinus');
      mask StyleString: edit,popup(8|6|5.3|5.2|5.1|4|3|2),edit,edit,edit,edit,edit,edit,edit,edit,edit,edit,popup(0|1|2),edit,checkbox
      mask CallbackString: |fm_block|||||||||||||fm_block
      mask Display:
      | plot(x+1.4,y,0.12*xs+1,0.15*ys-0.6)
      | color('blue')
      | plot(1.4+0.45*xg,0.3+0.45*yg)
  Syn4 : Subsystem  Tag=PSATblock  Description=Machines  Orientation=left  mask(Syn){p2_3_4q=[70000  20   60], p5q=3, p7_6q=[0.001  0*0.135], p8_9_10q=[1.79  0.22  0.18], p11_12q=[4.3  0.032], p13_14_15q=[1.715  0.4  0.215], p16_17q=[0.565  0.062], p18_19q=[2*3.93  2.00], p20_21q=[0.00  0.00], p22_23q=[1.00  1.00], p24q=0, p25_26q=[0 0], in=2, p27q=1, p28q=on}
      mask prompts: p2_3_4q "Power, voltage and frequency ratings [MVA, kV, Hz]"; p5q "Machine Dynamic Order"; p7_6q "resistance ra and leakage reactance xl [p.u. p.u.]"; p8_9_10q "d-axis reactances Xd, X'd X"d [p.u.,p.u.,p.u.]"; p11_12q "d-axis open circuit time constants T'd0 and T"d0 [s, s]"; p13_14_15q "q-axis reactances Xq, X'q, X"q [p.u.  p.u.  p.u.]"; p16_17q "q-axis open circuit time constants T'q0 and T"q0 [s s]"; p18_19q "Inertia (M = 2H) and Damping [s, p.u.]"; p20_21q "Speed and active power additional signals Kw and Kp [p.u., p.u.]"; p22_23q "Percentage of active and reactive powers at bus [p.u. p.u.]"; p24q "d-axis additional circuit leakage time constant Taa [s]"; p25_26q "Saturation coefficients S(1.0) and S(1.2)"; in "Number of input signals"; p27q "COI number"; p28q "Connected"
      mask help: This block defines a fourth order synchronous machine.
      mask init:
      | fm_inout
      | [x,y] = fm_draw('circle');
      | [xg,yg] = fm_draw('G');
      | [xs,ys] = fm_draw('sinus');
      mask StyleString: edit,popup(8|6|5.3|5.2|5.1|4|3|2),edit,edit,edit,edit,edit,edit,edit,edit,edit,edit,popup(0|1|2),edit,checkbox
      mask CallbackString: |fm_block|||||||||||||fm_block
      mask Display:
      | plot(x+1.4,y,0.12*xs+1,0.15*ys-0.6)
      | color('blue')
      | plot(1.4+0.45*xg,0.3+0.45*yg)
  Tg1 : Subsystem  Tag=PSATblock  Description=Controls  mask(Tg){p2q=1, p3q=1.00, p4q=0.04, p5q=100, p6q=0, p7q=20, p8q=0.2, p9q=0.2, p10q=0.2, p11q=0.2}
      mask prompts: p2q "Turbine governor type"; p3q "Reference speed [p.u.]"; p4q "Droop R [p.u./p.u.]"; p5q "Maximum torque [p.u.]"; p6q "Minimum torque [p.u.]"; p7q "Governor Time Constant Ts [s]"; p8q "Servo Time Constant Tc [s]"; p9q "Transient gain time constant T3 [s]"; p10q "Power fraction time constant T4 [s]"; p11q "Reheat time constant T5 [s]"
      mask help: This block defines a Turbine Governor.
      mask init:
      | [x,y] = fm_draw('G');
      mask Help:
      | This block defines  a Turbine Governor.
      | There are two kind of regulators:
      | 
      | Type 1:
      | 
      |      IEEE Model 4
      | 
      | Type 2:
      | 
      |      IEEE Model 1
      mask StyleString: popup(1|2),edit,edit,edit,edit,edit,edit,edit,edit,edit
      mask CallbackString: fm_block|||||||||
      mask Display:
      | plot([-1.8 2.8 2.8 -1.8 -1.8],[-1.5 -1.5 1.5 1.5 -1.5])
      | color('red')
      | plot([-0.5 -0.5],[-1 1],[-1.3 0.3],[1 1])
      | plot(1.4+x,y)
  Tg2 : Subsystem  Tag=PSATblock  Description=Controls  mask(Tg){p2q=1, p3q=1.00, p4q=0.04, p5q=100, p6q=0, p7q=20, p8q=0.2, p9q=0.2, p10q=0.2, p11q=0.2}
      mask prompts: p2q "Turbine governor type"; p3q "Reference speed [p.u.]"; p4q "Droop R [p.u./p.u.]"; p5q "Maximum torque [p.u.]"; p6q "Minimum torque [p.u.]"; p7q "Governor Time Constant Ts [s]"; p8q "Servo Time Constant Tc [s]"; p9q "Transient gain time constant T3 [s]"; p10q "Power fraction time constant T4 [s]"; p11q "Reheat time constant T5 [s]"
      mask help: This block defines a Turbine Governor.
      mask init:
      | [x,y] = fm_draw('G');
      mask Help:
      | This block defines  a Turbine Governor.
      | There are two kind of regulators:
      | 
      | Type 1:
      | 
      |      IEEE Model 4
      | 
      | Type 2:
      | 
      |      IEEE Model 1
      mask StyleString: popup(1|2),edit,edit,edit,edit,edit,edit,edit,edit,edit
      mask CallbackString: fm_block|||||||||
      mask Display:
      | plot([-1.8 2.8 2.8 -1.8 -1.8],[-1.5 -1.5 1.5 1.5 -1.5])
      | color('red')
      | plot([-0.5 -0.5],[-1 1],[-1.3 0.3],[1 1])
      | plot(1.4+x,y)
  Tg3 : Subsystem  Tag=PSATblock  Description=Controls  Orientation=left  mask(Tg){p2q=1, p3q=1.00, p4q=0.04, p5q=100, p6q=0, p7q=20, p8q=0.2, p9q=0.2, p10q=0.2, p11q=0.2}
      mask prompts: p2q "Turbine governor type"; p3q "Reference speed [p.u.]"; p4q "Droop R [p.u./p.u.]"; p5q "Maximum torque [p.u.]"; p6q "Minimum torque [p.u.]"; p7q "Governor Time Constant Ts [s]"; p8q "Servo Time Constant Tc [s]"; p9q "Transient gain time constant T3 [s]"; p10q "Power fraction time constant T4 [s]"; p11q "Reheat time constant T5 [s]"
      mask help: This block defines a Turbine Governor.
      mask init:
      | [x,y] = fm_draw('G');
      mask Help:
      | This block defines  a Turbine Governor.
      | There are two kind of regulators:
      | 
      | Type 1:
      | 
      |      IEEE Model 4
      | 
      | Type 2:
      | 
      |      IEEE Model 1
      mask StyleString: popup(1|2),edit,edit,edit,edit,edit,edit,edit,edit,edit
      mask CallbackString: fm_block|||||||||
      mask Display:
      | plot([-1.8 2.8 2.8 -1.8 -1.8],[-1.5 -1.5 1.5 1.5 -1.5])
      | color('red')
      | plot([-0.5 -0.5],[-1 1],[-1.3 0.3],[1 1])
      | plot(1.4+x,y)
  Tg4 : Subsystem  Tag=PSATblock  Description=Controls  Orientation=left  mask(Tg){p2q=1, p3q=1.00, p4q=0.04, p5q=100, p6q=0, p7q=20, p8q=0.2, p9q=0.2, p10q=0.2, p11q=0.2}
      mask prompts: p2q "Turbine governor type"; p3q "Reference speed [p.u.]"; p4q "Droop R [p.u./p.u.]"; p5q "Maximum torque [p.u.]"; p6q "Minimum torque [p.u.]"; p7q "Governor Time Constant Ts [s]"; p8q "Servo Time Constant Tc [s]"; p9q "Transient gain time constant T3 [s]"; p10q "Power fraction time constant T4 [s]"; p11q "Reheat time constant T5 [s]"
      mask help: This block defines a Turbine Governor.
      mask init:
      | [x,y] = fm_draw('G');
      mask Help:
      | This block defines  a Turbine Governor.
      | There are two kind of regulators:
      | 
      | Type 1:
      | 
      |      IEEE Model 4
      | 
      | Type 2:
      | 
      |      IEEE Model 1
      mask StyleString: popup(1|2),edit,edit,edit,edit,edit,edit,edit,edit,edit
      mask CallbackString: fm_block|||||||||
      mask Display:
      | plot([-1.8 2.8 2.8 -1.8 -1.8],[-1.5 -1.5 1.5 1.5 -1.5])
      | color('red')
      | plot([-0.5 -0.5],[-1 1],[-1.3 0.3],[1 1])
      | plot(1.4+x,y)
  Transf1 : PMComponent  Tag=PSATblock  Description=Power Flow  PhysicalDomain=psatdomain  LeftPortType=p1  RightPortType=p1  LConnTagsString=__newl0  RConnTagsString=__newr0  mask(Line){p3_4_5q=[100  20  60], p7q=20/400, p8q=0.00, p9q=0.0002, p13_14_15q=[0.0  0.0  0.0], p16q=on}
      mask prompts: p3_4_5q "Power, Voltage and Frequency Ratings [MVA, kV, Hz]"; p7q "Primary and secondary voltage ratio [kV/kV]"; p8q "Resistance [p.u.]"; p9q "Reactance [p.u.]"; p13_14_15q "Imax, Pmax and Smax [p.u., p.u., p.u.]"; p16q "Connected"
      mask help: This block defines a transformer.
      mask init:
      | [x,y] = fm_draw('circle');
      | [x1,y1] = fm_draw('1');
      | [x2,y2] = fm_draw('2');
      mask CallbackString: |||||fm_block
      mask Display:
      | plot(x,y,x+1.4,y,[-1 -1.3],[0 0],[2.4 2.7],[0 0])
      | color('green')
      | plot(-0.1+0.65*x1,0.65*y1)
      | plot(1.5+0.65*x2,0.65*y2)
  Transf2 : PMComponent  Tag=PSATblock  Description=Power Flow  PhysicalDomain=psatdomain  LeftPortType=p1  RightPortType=p1  LConnTagsString=__newl0  RConnTagsString=__newr0  mask(Line){p3_4_5q=[100  20  60], p7q=20/400, p8q=0, p9q=0.0066, p13_14_15q=[0.0  0.0  0.0], p16q=on}
      mask prompts: p3_4_5q "Power, Voltage and Frequency Ratings [MVA, kV, Hz]"; p7q "Primary and secondary voltage ratio [kV/kV]"; p8q "Resistance [p.u.]"; p9q "Reactance [p.u.]"; p13_14_15q "Imax, Pmax and Smax [p.u., p.u., p.u.]"; p16q "Connected"
      mask help: This block defines a transformer.
      mask init:
      | [x,y] = fm_draw('circle');
      | [x1,y1] = fm_draw('1');
      | [x2,y2] = fm_draw('2');
      mask CallbackString: |||||fm_block
      mask Display:
      | plot(x,y,x+1.4,y,[-1 -1.3],[0 0],[2.4 2.7],[0 0])
      | color('green')
      | plot(-0.1+0.65*x1,0.65*y1)
      | plot(1.5+0.65*x2,0.65*y2)
  Transf3 : PMComponent  Tag=PSATblock  Description=Power Flow  Orientation=left  PhysicalDomain=psatdomain  LeftPortType=p1  RightPortType=p1  LConnTagsString=__newl0  RConnTagsString=__newr0  mask(Line){p3_4_5q=[100  20  60], p7q=20/400, p8q=0, p9q=0.002, p13_14_15q=[0.0  0.0  0.0], p16q=on}
      mask prompts: p3_4_5q "Power, Voltage and Frequency Ratings [MVA, kV, Hz]"; p7q "Primary and secondary voltage ratio [kV/kV]"; p8q "Resistance [p.u.]"; p9q "Reactance [p.u.]"; p13_14_15q "Imax, Pmax and Smax [p.u., p.u., p.u.]"; p16q "Connected"
      mask help: This block defines a transformer.
      mask init:
      | [x,y] = fm_draw('circle');
      | [x1,y1] = fm_draw('1');
      | [x2,y2] = fm_draw('2');
      mask CallbackString: |||||fm_block
      mask Display:
      | plot(x,y,x+1.4,y,[-1 -1.3],[0 0],[2.4 2.7],[0 0])
      | color('green')
      | plot(-0.1+0.65*x1,0.65*y1)
      | plot(1.5+0.65*x2,0.65*y2)
  Transf4 : PMComponent  Tag=PSATblock  Description=Power Flow  Orientation=left  PhysicalDomain=psatdomain  LeftPortType=p1  RightPortType=p1  LConnTagsString=__newl0  RConnTagsString=__newr0  mask(Line){p3_4_5q=[100  20  60], p7q=20/400, p8q=0, p9q=0.000143, p13_14_15q=[0.0  0.0  0.0], p16q=on}
      mask prompts: p3_4_5q "Power, Voltage and Frequency Ratings [MVA, kV, Hz]"; p7q "Primary and secondary voltage ratio [kV/kV]"; p8q "Resistance [p.u.]"; p9q "Reactance [p.u.]"; p13_14_15q "Imax, Pmax and Smax [p.u., p.u., p.u.]"; p16q "Connected"
      mask help: This block defines a transformer.
      mask init:
      | [x,y] = fm_draw('circle');
      | [x1,y1] = fm_draw('1');
      | [x2,y2] = fm_draw('2');
      mask CallbackString: |||||fm_block
      mask Display:
      | plot(x,y,x+1.4,y,[-1 -1.3],[0 0],[2.4 2.7],[0 0])
      | color('green')
      | plot(-0.1+0.65*x1,0.65*y1)
      | plot(1.5+0.65*x2,0.65*y2)
  wires:
  Exc4/1(Out1) -> Syn4/1(in_1)
  Exc1/1(Out1) -> Syn1/1(in_1)
  Exc2/1(Out1) -> Syn2/1(in_1)
  Exc3/1(Out1) -> Syn3/1(in_1)
  Pss2/1(Out1) -> Exc2/1(in_1)
  Pss3/1(Out1) -> Exc3/1(in_1)
  Tg1/1(Out1) -> Syn1/2(in_2)
  Tg2/1(Out1) -> Syn2/2(in_2)
  Tg3/1(Out1) -> Syn3/2(in_2)
  Tg4/1(Out1) -> Syn4/2(in_2)
  connections:
  PV/RConn1 -- Bus1/LConn2
  Syn1/RConn1 -- Bus1/LConn1
  Bus1/RConn1 -- Transf1/LConn1
  Transf1/RConn1 -- Bus5/LConn1
  PQ/LConn1 -- Bus5/LConn2
  Bus5/RConn1 -- Line/LConn1
  Bus6/RConn2 -- Line1/LConn1
  Bus5/RConn2 -- Line2/LConn1
  Line2/RConn1 -- Bus6/RConn1
  Bus2/RConn1 -- Transf2/LConn1
  PV1/RConn1 -- Bus2/LConn2
  Syn2/RConn1 -- Bus2/LConn1
  Bus8/LConn1 -- PQ2/LConn1
  Transf3/RConn1 -- Bus8/RConn3
  Bus3/LConn1 -- Transf3/LConn1
  PV2/RConn1 -- Bus3/RConn2
  Syn3/RConn1 -- Bus3/RConn1
  Line6/LConn1 -- Bus8/RConn1
  Line5/LConn1 -- Bus8/RConn2
  Bus9/LConn2 -- Line5/RConn1
  Bus9/LConn1 -- Line6/RConn1
  Transf4/LConn1 -- Bus4/LConn1
  Slack/RConn1 -- Bus4/RConn2
  Syn4/RConn1 -- Bus4/RConn1
  Bus5/LConn3 -- Pl/LConn1
  Transf4/RConn1 -- Bus9/RConn1
  Bus9/RConn2 -- PQ3/LConn1
  Bus9/RConn3 -- Pl1/LConn1
  Transf2/RConn1 -- Bus6/LConn3
  Bus6/LConn2 -- PQ4/LConn1
  Line3/RConn1 -- Bus8/LConn3
  Line4/RConn1 -- Bus8/LConn4
  Bus6/LConn1 -- Pl2/LConn1
  Line4/LConn1 -- Bus7/RConn4
  Line3/LConn1 -- Bus7/RConn3
  Line1/RConn1 -- Bus7/LConn3
  Line/RConn1 -- Bus7/LConn1
  Bus8/LConn2 -- Pl3/LConn1
  Bus7/LConn2 -- Shunt1/LConn1
  PQ1/LConn1 -- Bus7/RConn1
  Pl4/LConn1 -- Bus7/RConn2
  Bus6/RConn3 -- Fault/LConn1
